simulink model "test1"  (R2018a)
settings: Solver=VariableStepAuto  StartTime=0.0  StopTime=10.0  RelTol=1e-3
libraries: powerlib x48, fl_lib x4
settings Model: Creator=u19ee  LastModifiedBy=u19ee

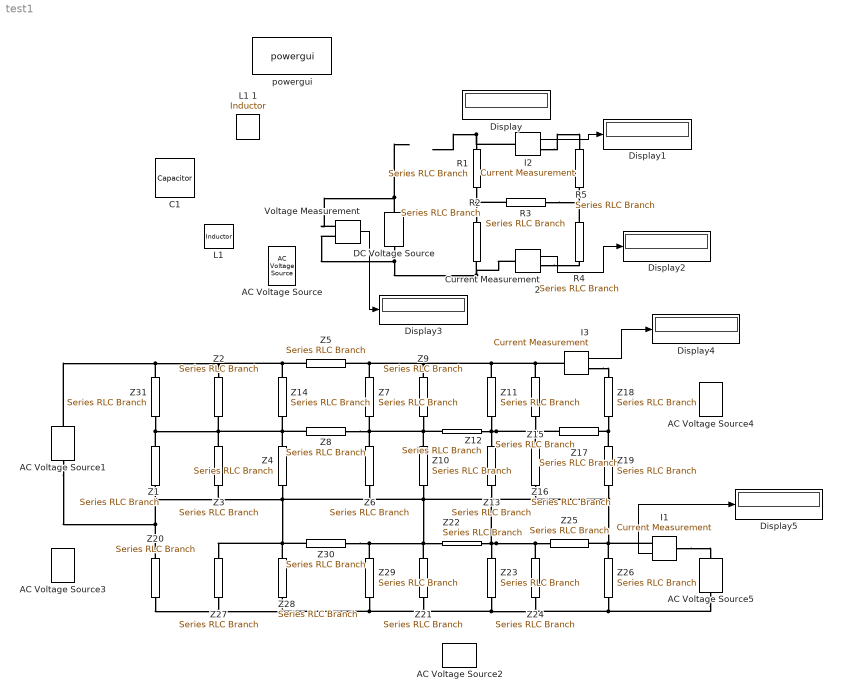
== system test1 ==
  AC Voltage Source : fl_lib/Electrical/Electrical Sources/AC Voltage Source  amp=1 V  shift=0 deg  frequency=60 Hz  omega=0 rad/s
  AC Voltage Source1 : powerlib/Electrical Sources/AC Voltage Source  Amplitude=100  Phase=0  Frequency=60  SampleTime=0  Measurements=None  BusType=swing  Pref=10e3  Qref=0  Qmin=-inf  Qmax=+inf
  AC Voltage Source2 : powerlib/Electrical Sources/AC Voltage Source  Amplitude=140  Phase=0  Frequency=60  SampleTime=0  Measurements=None  BusType=swing  Pref=10e3  Qref=0  Qmin=-inf  Qmax=+inf
  AC Voltage Source3 : powerlib/Electrical Sources/AC Voltage Source  Amplitude=120  Phase=0  Frequency=60  SampleTime=0  Measurements=None  BusType=swing  Pref=10e3  Qref=0  Qmin=-inf  Qmax=+inf
  AC Voltage Source4 : powerlib/Electrical Sources/AC Voltage Source  Amplitude=180  Phase=0  Frequency=60  SampleTime=0  Measurements=None  BusType=swing  Pref=10e3  Qref=0  Qmin=-inf  Qmax=+inf
  AC Voltage Source5 : powerlib/Electrical Sources/AC Voltage Source  Amplitude=160  Phase=0  Frequency=60  SampleTime=0  Measurements=None  BusType=swing  Pref=10e3  Qref=0  Qmin=-inf  Qmax=+inf
  C1 : fl_lib/Electrical/Electrical Elements/Capacitor  c=1e-6 F  r=1e-6 Ohm  g=0 1/Ohm  i_specify=off  i_priority=None  i=0 A  i_nominal_specify=off  i_nominal_unit=A  i_nominal_value=1  v_specify=off  v_priority=None  v=0 V  v_nominal_specify=off  v_nominal_unit=V  v_nominal_value=1  vc_specify=off  vc_priority=High  vc=0 V  vc_nominal_specify=off  vc_nominal_unit=V  vc_nominal_value=1
  Current Measurement2 : powerlib/Measurements/Current Measurement  PhasorSimulation=off  OutputType=Complex  PSBequivalent=0
  DC Voltage Source : powerlib/Electrical Sources/DC Voltage Source  Amplitude=10  Measurements=None
  Display{,1..5} (6 alike) : Display
  I1 : powerlib/Measurements/Current Measurement  PhasorSimulation=off  OutputType=Complex  PSBequivalent=0
  I2 : powerlib/Measurements/Current Measurement  PhasorSimulation=off  OutputType=Complex  PSBequivalent=0
  I3 : powerlib/Measurements/Current Measurement  PhasorSimulation=off  OutputType=Complex  PSBequivalent=0
  "L1 " : fl_lib/Electrical/Electrical Elements/Inductor  l=1e-6 H  r=0 Ohm  g=1e-9 1/Ohm  i_specify=off  i_priority=None  i=0 A  i_nominal_specify=off  i_nominal_unit=A  i_nominal_value=1  v_specify=off  v_priority=None  v=0 V  v_nominal_specify=off  v_nominal_unit=V  v_nominal_value=1  i_L_specify=off  i_L_priority=High  i_L=0 A  i_L_nominal_specify=off  i_L_nominal_unit=A  i_L_nominal_value=1
  L1 1 : fl_lib/Electrical/Electrical Elements/Inductor  l=1e-6 H  r=0 Ohm  g=1e-9 1/Ohm  i_specify=off  i_priority=None  i=0 A  i_nominal_specify=off  i_nominal_unit=A  i_nominal_value=1  v_specify=off  v_priority=None  v=0 V  v_nominal_specify=off  v_nominal_unit=V  v_nominal_value=1  i_L_specify=off  i_L_priority=High  i_L=0 A  i_L_nominal_specify=off  i_L_nominal_unit=A  i_L_nominal_value=1
  R1 : powerlib/Elements/Series RLC Branch  LConnTagsString=__new0  RConnTagsString=__new0  BranchType=R  Resistance=10  Inductance=0  SetiL0=off  InitialCurrent=0  Capacitance=0  Setx0=off  InitialVoltage=0  Measurements=None
  R2 : powerlib/Elements/Series RLC Branch  LConnTagsString=__new0  RConnTagsString=__new0  BranchType=R  Resistance=30  Inductance=0  SetiL0=off  InitialCurrent=0  Capacitance=0  Setx0=off  InitialVoltage=0  Measurements=None
  R3 : powerlib/Elements/Series RLC Branch  LConnTagsString=__new0  RConnTagsString=__new0  BranchType=R  Resistance=5  Inductance=0  SetiL0=off  InitialCurrent=0  Capacitance=0  Setx0=off  InitialVoltage=0  Measurements=None
  R4 : powerlib/Elements/Series RLC Branch  LConnTagsString=__new0  RConnTagsString=__new0  BranchType=R  Resistance=30  Inductance=0  SetiL0=off  InitialCurrent=0  Capacitance=0  Setx0=off  InitialVoltage=0  Measurements=None
  R5 : powerlib/Elements/Series RLC Branch  LConnTagsString=__new0  RConnTagsString=__new0  BranchType=R  Resistance=15  Inductance=0  SetiL0=off  InitialCurrent=0  Capacitance=0  Setx0=off  InitialVoltage=0  Measurements=None
  Voltage Measurement : powerlib/Measurements/Voltage Measurement  PhasorSimulation=off  OutputType=Magnitude  PSBequivalent=0
  Z1 : powerlib/Elements/Series RLC Branch  LConnTagsString=__new0  RConnTagsString=__new0  BranchType=RLC  Resistance=1671  Inductance=0.425415919583203  SetiL0=off  InitialCurrent=0  Capacitance=419  Setx0=off  InitialVoltage=0  Measurements=None
  Z10 : powerlib/Elements/Series RLC Branch  LConnTagsString=__new0  RConnTagsString=__new0  BranchType=RLC  Resistance=1892  Inductance=0.683628887062374  SetiL0=off  InitialCurrent=0  Capacitance=321  Setx0=off  InitialVoltage=0  Measurements=None
  Z11 : powerlib/Elements/Series RLC Branch  LConnTagsString=__new0  RConnTagsString=__new0  BranchType=RLC  Resistance=517  Inductance=0.824401118170665  SetiL0=off  InitialCurrent=0  Capacitance=487  Setx0=off  InitialVoltage=0  Measurements=None
  Z12 : powerlib/Elements/Series RLC Branch  LConnTagsString=__new0  RConnTagsString=__new0  BranchType=RLC  Resistance=40  Inductance=0.447234580788824  SetiL0=off  InitialCurrent=0  Capacitance=173  Setx0=off  InitialVoltage=0  Measurements=None
  Z13 : powerlib/Elements/Series RLC Branch  LConnTagsString=__new0  RConnTagsString=__new0  BranchType=RLC  Resistance=440  Inductance=0.266531217060233  SetiL0=off  InitialCurrent=0  Capacitance=394  Setx0=off  InitialVoltage=0  Measurements=None
  Z14 : powerlib/Elements/Series RLC Branch  LConnTagsString=__new0  RConnTagsString=__new0  BranchType=RLC  Resistance=2679  Inductance=0.431435725807843  SetiL0=off  InitialCurrent=0  Capacitance=299  Setx0=off  InitialVoltage=0  Measurements=None
  Z15 : powerlib/Elements/Series RLC Branch  LConnTagsString=__new0  RConnTagsString=__new0  BranchType=RLC  Resistance=3111  Inductance=0.317938098929446  SetiL0=off  InitialCurrent=0  Capacitance=287  Setx0=off  InitialVoltage=0  Measurements=None
  Z16 : powerlib/Elements/Series RLC Branch  LConnTagsString=__new0  RConnTagsString=__new0  BranchType=RLC  Resistance=2309  Inductance=0.848265575156744  SetiL0=off  InitialCurrent=0  Capacitance=496  Setx0=off  InitialVoltage=0  Measurements=None
  Z17 : powerlib/Elements/Series RLC Branch  LConnTagsString=__new0  RConnTagsString=__new0  BranchType=RLC  Resistance=1971  Inductance=0.792156483965612  SetiL0=off  InitialCurrent=0  Capacitance=209  Setx0=off  InitialVoltage=0  Measurements=None
  Z18 : powerlib/Elements/Series RLC Branch  LConnTagsString=__new0  RConnTagsString=__new0  BranchType=RLC  Resistance=724  Inductance=0.274968825462546  SetiL0=off  InitialCurrent=0  Capacitance=452  Setx0=off  InitialVoltage=0  Measurements=None
  Z19 : powerlib/Elements/Series RLC Branch  LConnTagsString=__new0  RConnTagsString=__new0  BranchType=RLC  Resistance=1942  Inductance=0.948490106350500  SetiL0=off  InitialCurrent=0  Capacitance=456  Setx0=off  InitialVoltage=0  Measurements=None
  Z2 : powerlib/Elements/Series RLC Branch  LConnTagsString=__new0  RConnTagsString=__new0  BranchType=RLC  Resistance=213  Inductance=0.181839163086784  SetiL0=off  InitialCurrent=0  Capacitance=88  Setx0=off  InitialVoltage=0  Measurements=None
  Z20 : powerlib/Elements/Series RLC Branch  LConnTagsString=__new0  RConnTagsString=__new0  BranchType=RLC  Resistance=2059  Inductance=0.111874866579224  SetiL0=off  InitialCurrent=0  Capacitance=64  Setx0=off  InitialVoltage=0  Measurements=None
  Z21 : powerlib/Elements/Series RLC Branch  LConnTagsString=__new0  RConnTagsString=__new0  BranchType=RLC  Resistance=380  Inductance=0.815685022889823  SetiL0=off  InitialCurrent=0  Capacitance=471  Setx0=off  InitialVoltage=0  Measurements=None
  Z22 : powerlib/Elements/Series RLC Branch  LConnTagsString=__new0  RConnTagsString=__new0  BranchType=RLC  Resistance=2061  Inductance=0.963238421923673  SetiL0=off  InitialCurrent=0  Capacitance=44  Setx0=off  InitialVoltage=0  Measurements=None
  Z23 : powerlib/Elements/Series RLC Branch  LConnTagsString=__new0  RConnTagsString=__new0  BranchType=RLC  Resistance=82  Inductance=0.996327734605249  SetiL0=off  InitialCurrent=0  Capacitance=154  Setx0=off  InitialVoltage=0  Measurements=None
  Z24 : powerlib/Elements/Series RLC Branch  LConnTagsString=__new0  RConnTagsString=__new0  BranchType=RLC  Resistance=801  Inductance=0.039983622190244  SetiL0=off  InitialCurrent=0  Capacitance=385  Setx0=off  InitialVoltage=0  Measurements=None
  Z25 : powerlib/Elements/Series RLC Branch  LConnTagsString=__new0  RConnTagsString=__new0  BranchType=RLC  Resistance=1554  Inductance=0.828999333485437  SetiL0=off  InitialCurrent=0  Capacitance=233  Setx0=off  InitialVoltage=0  Measurements=None
  Z26 : powerlib/Elements/Series RLC Branch  LConnTagsString=__new0  RConnTagsString=__new0  BranchType=RLC  Resistance=3010  Inductance=0.603011473965450  SetiL0=off  InitialCurrent=0  Capacitance=462  Setx0=off  InitialVoltage=0  Measurements=None
  Z27 : powerlib/Elements/Series RLC Branch  LConnTagsString=__new0  RConnTagsString=__new0  BranchType=RLC  Resistance=472  Inductance=0.861358788047135  SetiL0=off  InitialCurrent=0  Capacitance=92  Setx0=off  InitialVoltage=0  Measurements=None
  Z28 : powerlib/Elements/Series RLC Branch  LConnTagsString=__new0  RConnTagsString=__new0  BranchType=RLC  Resistance=1006  Inductance=0.509809229215785  SetiL0=off  InitialCurrent=0  Capacitance=135  Setx0=off  InitialVoltage=0  Measurements=None
  Z29 : powerlib/Elements/Series RLC Branch  LConnTagsString=__new0  RConnTagsString=__new0  BranchType=RLC  Resistance=3010  Inductance=0.603011473965450  SetiL0=off  InitialCurrent=0  Capacitance=462  Setx0=off  InitialVoltage=0  Measurements=None
  Z3 : powerlib/Elements/Series RLC Branch  LConnTagsString=__new0  RConnTagsString=__new0  BranchType=RLC  Resistance=1805  Inductance=0.885376918636421  SetiL0=off  InitialCurrent=0  Capacitance=360  Setx0=off  InitialVoltage=0  Measurements=None
  Z30 : powerlib/Elements/Series RLC Branch  LConnTagsString=__new0  RConnTagsString=__new0  BranchType=RLC  Resistance=472  Inductance=0.861358788047135  SetiL0=off  InitialCurrent=0  Capacitance=92  Setx0=off  InitialVoltage=0  Measurements=None
  Z31 : powerlib/Elements/Series RLC Branch  LConnTagsString=__new0  RConnTagsString=__new0  BranchType=RLC  Resistance=1006  Inductance=0.509809229215785  SetiL0=off  InitialCurrent=0  Capacitance=135  Setx0=off  InitialVoltage=0  Measurements=None
  Z4 : powerlib/Elements/Series RLC Branch  LConnTagsString=__new0  RConnTagsString=__new0  BranchType=RLC  Resistance=281  Inductance=0.992479819054851  SetiL0=off  InitialCurrent=0  Capacitance=158  Setx0=off  InitialVoltage=0  Measurements=None
  Z5 : powerlib/Elements/Series RLC Branch  LConnTagsString=__new0  RConnTagsString=__new0  BranchType=RLC  Resistance=2720  Inductance=0.806171764514278  SetiL0=off  InitialCurrent=0  Capacitance=152  Setx0=off  InitialVoltage=0  Measurements=None
  Z6 : powerlib/Elements/Series RLC Branch  LConnTagsString=__new0  RConnTagsString=__new0  BranchType=RLC  Resistance=2632  Inductance=0.394658562414268  SetiL0=off  InitialCurrent=0  Capacitance=142  Setx0=off  InitialVoltage=0  Measurements=None
  Z7 : powerlib/Elements/Series RLC Branch  LConnTagsString=__new0  RConnTagsString=__new0  BranchType=RLC  Resistance=1644  Inductance=0.071648249156369  SetiL0=off  InitialCurrent=0  Capacitance=262  Setx0=off  InitialVoltage=0  Measurements=None
  Z8 : powerlib/Elements/Series RLC Branch  LConnTagsString=__new0  RConnTagsString=__new0  BranchType=RLC  Resistance=2151  Inductance=0.522075737663986  SetiL0=off  InitialCurrent=0  Capacitance=288  Setx0=off  InitialVoltage=0  Measurements=None
  Z9 : powerlib/Elements/Series RLC Branch  LConnTagsString=__new0  RConnTagsString=__new0  BranchType=RLC  Resistance=102  Inductance=0.100900315968770  SetiL0=off  InitialCurrent=0  Capacitance=422  Setx0=off  InitialVoltage=0  Measurements=None
  powergui : powerlib/powergui  Priority=1  SimulationMode=Continuous  SampleTime=50e-6  frequency=60  Iterations=50  frequencyindice=60  Pbase=100e6  ErrMax=1e-4  UnitsV=kV  UnitsW=MW  buscounter=0  FunctionMessages=off  echomessages=off  EnableUseOfTLC=off  CurrentSourceSwitches=off  DisableSnubberDevices=off  DisableRonSwitches=off  DisableVfSwitches=off  DisplayEquations=off  SolverType=Tustin/Backward Euler (TBE)  Interpol=off  ExternalGateDelay=off  methode=off  Ts=100  x0status=blocks  SPID=on  SwTol=0  HookPort=off  RestoreLinks=warning  ResistiveCurrentMeasurement=off  Frange=[0:2:500]  Ylog=off  Xlog=on  ShowGrid=off  save=off  variable=ZData  structure=0  ZoomFFT=off  StartTime=0.0  cycles=1  DisplayStyle=1  fundamental=60  FreqAxis=off  MaxFrequency=1000  frequencyindicesteady=1  RmsSteady=1  display=off
  wires:
  ? -> Display/1
  Voltage Measurement/1 -> Display3/1
  Current Measurement2/1 -> Display2/1
  I2/1 -> Display1/1
  I3/1 -> Display4/1
  I1/1 -> Display5/1
  connections:
  DC Voltage Source/RConn1 -- Voltage Measurement/LConn1
  R1/RConn1 -- R3/RConn1 -- R2/LConn1
  R3/LConn1 -- R4/LConn1 -- R5/RConn1
  I2/LConn1 -- R1/LConn1
  DC Voltage Source/LConn1 -- Voltage Measurement/LConn2 -- Current Measurement2/LConn1 -- R2/RConn1
  I2/RConn1 -- R5/LConn1
  Current Measurement2/RConn1 -- R4/RConn1
  Z4/LConn1 -- Z8/RConn1 -- Z31/RConn1 -- Z1/LConn1 -- Z3/LConn1 -- Z2/RConn1 -- Z14/RConn1
  Z14/LConn1 -- AC Voltage Source1/RConn1 -- Z31/LConn1 -- Z2/LConn1 -- Z5/RConn1
  Z8/LConn1 -- Z12/RConn1 -- Z10/LConn1 -- Z9/RConn1 -- Z6/LConn1 -- Z7/RConn1
  Z7/LConn1 -- I3/LConn1 -- Z15/LConn1 -- Z11/LConn1 -- Z9/LConn1 -- Z5/LConn1
  Z12/LConn1 -- Z17/RConn1 -- Z16/LConn1 -- Z15/RConn1 -- Z11/RConn1 -- Z13/LConn1
  Z18/LConn1 -- Z19/RConn1 -- Z17/LConn1
  AC Voltage Source5/LConn1 -- Z28/RConn1 -- Z20/RConn1 -- Z27/RConn1 -- Z29/RConn1 -- Z21/RConn1 -- Z23/RConn1 -- Z24/RConn1 -- Z26/LConn1
  Z20/LConn1 -- AC Voltage Source1/LConn1 -- Z3/RConn1 -- Z4/RConn1 -- Z28/LConn1 -- Z27/LConn1 -- Z30/RConn1 -- Z6/RConn1 -- Z10/RConn1 -- Z30/LConn1 -- Z29/LConn1 -- Z22/RConn1 -- Z21/LConn1 -- Z13/RConn1 -- Z24/LConn1 -- Z25/RConn1 -- Z22/LConn1 -- Z23/LConn1 -- I1/RConn1 -- Z25/LConn1 -- Z26/RConn1 -- Z19/LConn1 -- Z16/RConn1 -- Z1/RConn1
  I1/LConn1 -- AC Voltage Source5/RConn1
  I3/RConn1 -- Z18/RConn1
